simulink model "c6_p8x"  (Simulink 7.4)
settings: Solver=ode45  StartTime=0.0  StopTime=10e-6  MaxStep=0.1e-9  RelTol=1e-3
StopFcn:
  | plot_spar(spar)
undefined symbols (not defined in the file or in its folder): magnitude
libraries: powerlib x41, dspindex x12, dspsigops x6, dspbuff3 x4, dspxfrm3 x4, dsparch3 x4, dsparch4 x4, dspsnks4 x2, dspmtrx3 x2, simulink x1
settings Model: Creator=dbenson  LastModifiedBy=Dick
settings OptimizationCC: InlineInvariantSignals=on  InitFltsAndDblsToZero=on
settings DebuggingCC: SaveWithParameterizedLinksMsg=none  SignalResolutionControl=TryResolveAllWithWarning  MultiTaskDSMMsg=warning  MultiTaskCondExecSysMsg=none  StrictBusMsg=None
settings RTWCC: IncludeERTFirstTime=on
settings GRTTargetCC: TargetFcnLib=ansi_tfl_tmw.mat

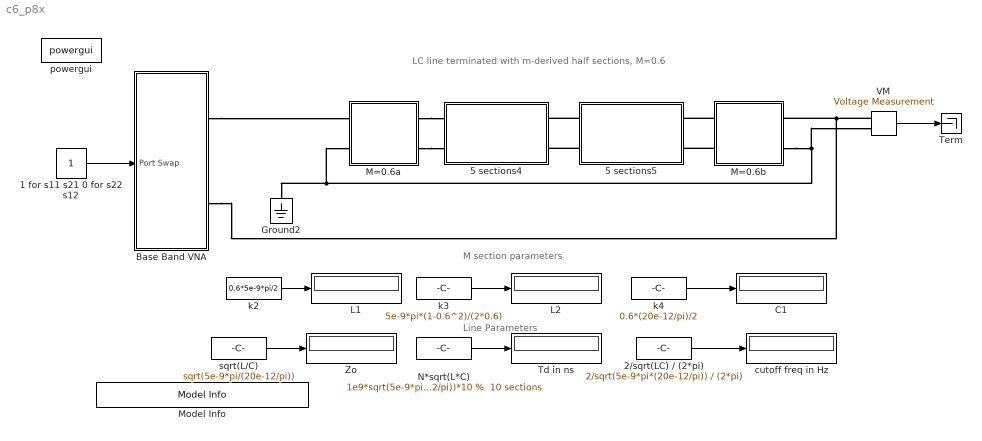
== system c6_p8x ==
  note: LC line terminated with m-derived half sections, M=0.6
  note: Line Parameters
  note: M section parameters
  1 for s11 s21 0 for s22 s12 : Constant  OutDataType=fixdt(1, 16)  OutScaling=2^0
  2/sqrt(LC) / (2*pi) : Constant  Value=2/sqrt(5e-9*pi*(20e-12/pi)) / (2*pi)  OutDataType=sfix(16)  OutScaling=2^0
  5 sections4 : Subsystem
  5 sections5 : Subsystem
  Base Band VNA : Subsystem  Description=Spectrum Analyzer  mask{BW=1e9, Frame_Size=512}
      mask prompts: BW "Bandwidth"; Frame_Size "FFT SIze (256,512,1024 etc)"
  C1 : Display
  Ground2 : powerlib/Elements/Ground  DialogController=POWERSYS.PowerSysDialog  PhysicalDomain=powersysdomain  SubClassName=unknown  LeftPortType=p1  RightPortType=p1  LConnTagsString=a
  L1 : Display
  L2 : Display
  M=0.6a : Subsystem
  M=0.6b : Subsystem
  Model Info : simulink/Model-Wide Utilities/Model Info  SystemSampleTime=-1  InitialBlockCM=None  BlockCM=None  Frame=on  DisplayStringWithTags=Copywrite 2005-2010 The MathWorks, Inc.  HorizontalTextAlignment=Center  LeftAlignmentValue=0.5  SourceBlockDiagram=c6_p8x  TagMaxNumber=20
  N*sqrt(L*C) : Constant  Value="1e9*sqrt(5e-9*pi*(20e-12/pi))*10 %  10 sections"  OutDataType=sfix(16)  OutScaling=2^0
  Td in ns : Display
  Term : Terminator
  VM : powerlib/Measurements/Voltage Measurement  DialogController=POWERSYS.PowerSysDialog  SystemSampleTime=-1  PhasorSimulation=off  OutputType=Complex  PSBequivalent=0
  Zo : Display
  cutoff freq in Hz : Display
  k2 : Constant  Value=0.6*5e-9*pi/2  OutDataType=sfix(16)  OutScaling=2^0
  k3 : Constant  Value=5e-9*pi*(1-0.6^2)/(2*0.6)  OutDataType=sfix(16)  OutScaling=2^0
  k4 : Constant  Value=0.6*(20e-12/pi)/2  OutDataType=sfix(16)  OutScaling=2^0
  powergui : powerlib/powergui  SystemSampleTime=-1  SimulationMode=Continuous  SampleTime=50e-6  frequency=60  SPID=off  DisableSnubberDevices=off  DisableRonSwitches=off  DisableVfSwitches=off  SwTol=0  Interpol=off  frequencyindice=0  echomessages=off  HookPort=off  DisplayEquations=off  FunctionMessages=off  EnableUseOfTLC=off  x0status=blocks  RestoreLinks=warning  Frange=[0:2:500]  Ylog=off  Xlog=on  ShowGrid=off  save=off  variable=ZData  ZoomFFT=on  StartTime=0.0  cycles=1  DisplayStyle=1  fundamental=60  FreqAxis=off  MaxFrequency=1000  frequencyindicesteady=1  RmsSteady=1  display=off  Ts=0  methode=off
  sqrt(L/C) : Constant  Value=sqrt(5e-9*pi/(20e-12/pi))  OutDataType=sfix(16)  OutScaling=2^0
  wires:
  sqrt(L/C)/1 -> Zo/1
  N*sqrt(L*C)/1 -> Td in ns/1
  k2/1 -> L1/1
  k3/1 -> L2/1
  k4/1 -> C1/1
  2/sqrt(LC) / (2*pi)/1 -> cutoff freq in Hz/1
  VM/1 -> Term/1
  1 for s11 s21 0 for s22 s12/1 -> Base Band VNA/1(Port Swap)
  connections:
  VM/LConn1 -- M=0.6b/RConn1 -- Base Band VNA/RConn2
  M=0.6a/RConn2 -- 5 sections4/LConn2
  5 sections5/LConn1 -- 5 sections4/RConn1
  5 sections5/LConn2 -- 5 sections4/RConn2
  M=0.6b/LConn1 -- 5 sections5/RConn1
  M=0.6b/LConn2 -- 5 sections5/RConn2
  M=0.6a/RConn1 -- 5 sections4/LConn1
  M=0.6b/RConn2 -- Ground2/LConn1 -- M=0.6a/LConn2 -- VM/LConn2
  Base Band VNA/RConn1 -- M=0.6a/LConn1

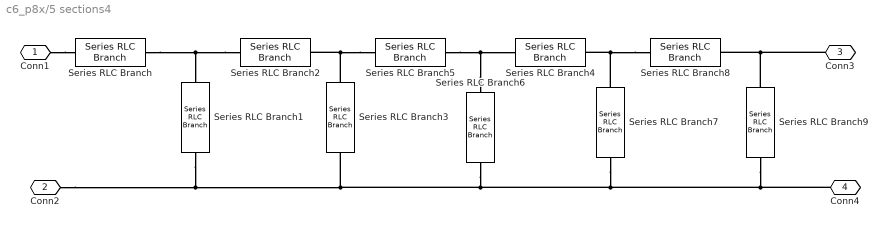
== system c6_p8x/5 sections4 ==
  Series RLC Branch{,2,4..5,8} (5 alike) : powerlib/Elements/Series RLC Branch  DialogController=POWERSYS.PowerSysDialog  PhysicalDomain=powersysdomain  SubClassName=unknown  LeftPortType=p1  RightPortType=p1  LConnTagsString=__new0  RConnTagsString=__new0  BranchType=L  Resistance=1.0  Inductance=5*pi*1e-9  SetiL0=off  InitialCurrent=0  Capacitance=1.0  Setx0=off  InitialVoltage=0  Measurements=None
  Series RLC Branch{1,3,6..7,9} (5 alike) : powerlib/Elements/Series RLC Branch  DialogController=POWERSYS.PowerSysDialog  PhysicalDomain=powersysdomain  SubClassName=unknown  LeftPortType=p1  RightPortType=p1  LConnTagsString=__new0  RConnTagsString=__new0  BranchType=C  Resistance=1.0  Inductance=1.0  SetiL0=off  InitialCurrent=0  Capacitance=20e-12/pi  Setx0=off  InitialVoltage=0  Measurements=None
  Conn1 : PMIOPort  Port=1  Side=Left
  Conn2 : PMIOPort  Port=2  Side=Left
  Conn3 : PMIOPort  Port=3  Side=Right
  Conn4 : PMIOPort  Port=4  Side=Right
  connections:
  Conn1/RConn1 -- Series RLC Branch/LConn1
  Conn3/RConn1 -- Series RLC Branch8/RConn1 -- Series RLC Branch9/LConn1
  Series RLC Branch8/LConn1 -- Series RLC Branch4/RConn1 -- Series RLC Branch7/LConn1
  Series RLC Branch6/LConn1 -- Series RLC Branch4/LConn1 -- Series RLC Branch5/RConn1
  Series RLC Branch5/LConn1 -- Series RLC Branch2/RConn1 -- Series RLC Branch3/LConn1
  Series RLC Branch7/RConn1 -- Conn4/RConn1 -- Series RLC Branch9/RConn1 -- Conn2/RConn1 -- Series RLC Branch1/RConn1 -- Series RLC Branch3/RConn1 -- Series RLC Branch6/RConn1
  Series RLC Branch2/LConn1 -- Series RLC Branch1/LConn1 -- Series RLC Branch/RConn1

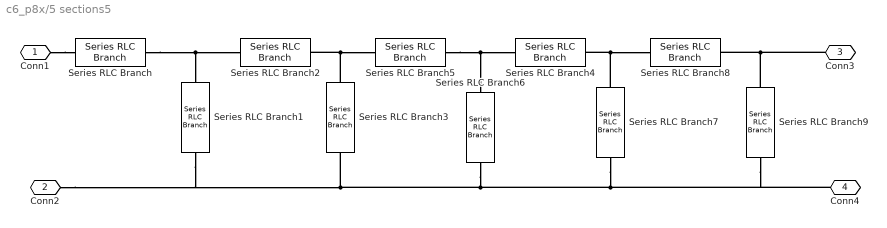
== system c6_p8x/5 sections5 ==
  Series RLC Branch{,2,4..5,8} (5 alike) : powerlib/Elements/Series RLC Branch  DialogController=POWERSYS.PowerSysDialog  PhysicalDomain=powersysdomain  SubClassName=unknown  LeftPortType=p1  RightPortType=p1  LConnTagsString=__new0  RConnTagsString=__new0  BranchType=L  Resistance=1.0  Inductance=5*pi*1e-9  SetiL0=off  InitialCurrent=0  Capacitance=1.0  Setx0=off  InitialVoltage=0  Measurements=None
  Series RLC Branch{1,3,6..7,9} (5 alike) : powerlib/Elements/Series RLC Branch  DialogController=POWERSYS.PowerSysDialog  PhysicalDomain=powersysdomain  SubClassName=unknown  LeftPortType=p1  RightPortType=p1  LConnTagsString=__new0  RConnTagsString=__new0  BranchType=C  Resistance=1.0  Inductance=1.0  SetiL0=off  InitialCurrent=0  Capacitance=20e-12/pi  Setx0=off  InitialVoltage=0  Measurements=None
  Conn1 : PMIOPort  Port=1  Side=Left
  Conn2 : PMIOPort  Port=2  Side=Left
  Conn3 : PMIOPort  Port=3  Side=Right
  Conn4 : PMIOPort  Port=4  Side=Right
  connections:
  Series RLC Branch/RConn1 -- Series RLC Branch1/LConn1 -- Series RLC Branch2/LConn1
  Series RLC Branch6/RConn1 -- Series RLC Branch3/RConn1 -- Series RLC Branch1/RConn1 -- Conn2/RConn1 -- Series RLC Branch9/RConn1 -- Conn4/RConn1 -- Series RLC Branch7/RConn1
  Series RLC Branch3/LConn1 -- Series RLC Branch2/RConn1 -- Series RLC Branch5/LConn1
  Series RLC Branch5/RConn1 -- Series RLC Branch4/LConn1 -- Series RLC Branch6/LConn1
  Series RLC Branch7/LConn1 -- Series RLC Branch4/RConn1 -- Series RLC Branch8/LConn1
  Series RLC Branch9/LConn1 -- Series RLC Branch8/RConn1 -- Conn3/RConn1
  Conn1/RConn1 -- Series RLC Branch/LConn1

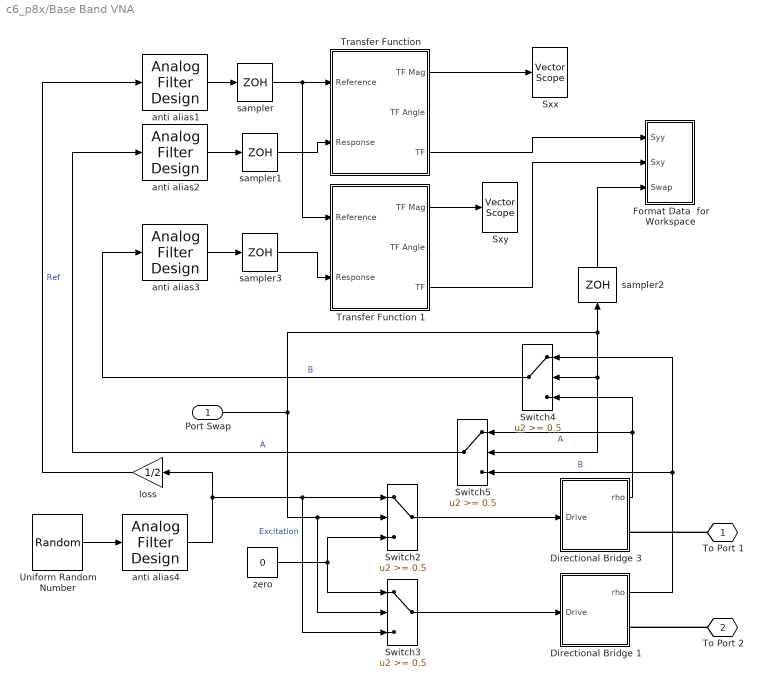
== system c6_p8x/Base Band VNA ==
  Port Swap : Inport  OutDataType=sfix(16)  OutScaling=2^0
  Directional Bridge 1 : Subsystem  mask{Zo=50}
      mask prompts: Zo "Zo="
  Directional Bridge 3 : Subsystem  mask{Zo=50}
      mask prompts: Zo "Zo="
  Format Data  for Workspace : Subsystem
  Switch{2..5} (4 alike) : Switch  Threshold=0.5  SaturateOnIntegerOverflow=on
  Sxx : dspsnks4/Vector Scope  DialogController=dspdialog.VectorScope  DialogControllerArgs=DataTag0  ScopeProperties=on  Domain=Frequency  HorizSpan=1  DisplayProperties=off  AxisGrid=on  Memory=off  FrameNumber=on  AxisLegend=off  AxisZoom=off  OpenScopeAtSimStart=on  OpenScopeImmediately=off  FigPos=[396 210 335 234]  AxisProperties=off  XUnits=Hertz  XRange=[0...Fs/2]  InheritXIncr=off  XIncr=1/(2.56*BW)  XLabel=Time  XLimit=Auto  XMin=0  XMax=1  XStart=0  YUnits=dB  YLabel=Amplitude  LineProperties=off  XAxisParamsVer=6.9
      settings: YMin=-30  YMax=25
  Sxy : dspsnks4/Vector Scope  DialogController=dspdialog.VectorScope  DialogControllerArgs=DataTag1  ScopeProperties=on  Domain=Frequency  HorizSpan=1  DisplayProperties=off  AxisGrid=on  Memory=off  FrameNumber=on  AxisLegend=off  AxisZoom=off  OpenScopeAtSimStart=on  OpenScopeImmediately=off  FigPos=[24 215 357 231]  AxisProperties=off  XUnits=Hertz  XRange=[0...Fs/2]  InheritXIncr=off  XIncr=1/(2.56*BW)  XLabel=Time  XLimit=Auto  XMin=0  XMax=1  XStart=0  YUnits=dB  YLabel=Amplitude  LineProperties=off  XAxisParamsVer=6.9
      settings: YMin=-30  YMax=25
  "Transfer Function " : Subsystem  mask{NFFT=Frame_Size, Navg=100, pcnt=100, unwrap_flag=on}
      mask prompts: NFFT "FFT length (power of 2):"; Navg "Spectral Averaging Factor (>=1):"; pcnt "Percentage of  Alias Free Data  (<=100)"; unwrap_flag "Unwrap Phase"
      mask Display: disp('Transfer Function \n Estimation (v2.0) ')
  Transfer Function 1 : Subsystem  mask{NFFT=Frame_Size, Navg=100, pcnt=100, unwrap_flag=on}
      mask prompts: NFFT "FFT length (power of 2):"; Navg "Spectral Averaging Factor (>=1):"; pcnt "Percentage of  Alias Free Data  (<=100)"; unwrap_flag "Unwrap Phase"
      mask Display: disp('Transfer Function \n Estimation (v2.0) ')
  Uniform Random Number : UniformRandomNumber  SampleTime=1/(2.56*BW)
  anti alias{1..4} (4 alike) : dsparch4/Analog Filter Design  method=Elliptic  filttype=Lowpass  N=8  Wlo=BW*2*pi  Whi=80  Rp=2  Rs=100
  loss : Gain  Gain=1/2  ParameterDataType=sfix(16)  ParameterScaling=2^0  OutDataType=sfix(16)  OutScaling=2^0  SaturateOnIntegerOverflow=on  OutDataTypeStr=Inherit: Same as input  ParamDataTypeStr=Inherit: Same as input
  sampler : ZeroOrderHold  SampleTime=1/(2.56*BW)
  sampler1 : ZeroOrderHold  SampleTime=1/(2.56*BW)
  sampler2 : ZeroOrderHold  SampleTime=256/(2.56*BW)
  sampler3 : ZeroOrderHold  SampleTime=1/(2.56*BW)
  zero : Constant  Value=0  OutDataType=sfix(16)  OutScaling=2^0
  To Port 1 : PMIOPort  Tag=PMCPort  Port=1  Side=Right
  To Port 2 : PMIOPort  Tag=PMCPort  Port=2  Side=Right
  wires:
  sampler/1 -> "Transfer Function "/1(Reference), Transfer Function 1/1(Reference)
  anti alias1/1 -> sampler/1
  anti alias2/1 -> sampler1/1
  Uniform Random Number/1 -> anti alias4/1
  anti alias3/1 -> sampler3/1
  sampler3/1 -> Transfer Function 1/2(Response)
  anti alias4/1 -> loss/1, Switch3/3, Switch2/1  "Excitation"
  loss/1 -> anti alias1/1  "Ref"
  Port Swap/1 -> Switch3/2, Switch2/2, Switch4/2, Switch5/2, sampler2/1
  zero/1 -> Switch2/3, Switch3/1
  Switch2/1 -> Directional Bridge 3/1(Drive)
  Switch3/1 -> Directional Bridge 1/1(Drive)
  Switch5/1 -> anti alias2/1  "A"
  Switch4/1 -> anti alias3/1  "B"
  Directional Bridge 3/1(rho) -> Switch4/3, Switch5/1  "A"
  Directional Bridge 1/1(rho) -> Switch5/3, Switch4/1  "B"
  sampler1/1 -> "Transfer Function "/2(Response)
  "Transfer Function "/1(TF Mag) -> Sxx/1
  Transfer Function 1/3("TF ") -> Format Data  for Workspace/2(Sxy)
  Transfer Function 1/1(TF Mag) -> Sxy/1
  "Transfer Function "/3("TF ") -> Format Data  for Workspace/1(Syy)
  sampler2/1 -> Format Data  for Workspace/3(Swap)
  connections:
  To Port 1/RConn1 -- Directional Bridge 3/RConn1
  To Port 2/RConn1 -- Directional Bridge 1/RConn1

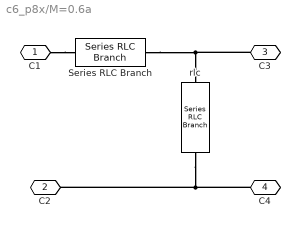
== system c6_p8x/M=0.6a ==
  Series RLC Branch : powerlib/Elements/Series RLC Branch  DialogController=POWERSYS.PowerSysDialog  PhysicalDomain=powersysdomain  SubClassName=unknown  LeftPortType=p1  RightPortType=p1  LConnTagsString=__new0  RConnTagsString=__new0  BranchType=L  Resistance=1.0  Inductance=4.712e-9  SetiL0=off  InitialCurrent=0  Capacitance=1.0  Setx0=off  InitialVoltage=0  Measurements=None
  rlc : powerlib/Elements/Series RLC Branch  DialogController=POWERSYS.PowerSysDialog  PhysicalDomain=powersysdomain  SubClassName=unknown  LeftPortType=p1  RightPortType=p1  LConnTagsString=__new0  RConnTagsString=__new0  BranchType=LC  Resistance=1.0  Inductance=8.378e-9  SetiL0=off  InitialCurrent=0  Capacitance=1.91e-12  Setx0=off  InitialVoltage=0  Measurements=None
  C1 : PMIOPort  Port=1  Side=Left
  C2 : PMIOPort  Port=2  Side=Left
  C3 : PMIOPort  Port=3  Side=Right
  C4 : PMIOPort  Port=4  Side=Right
  connections:
  C3/RConn1 -- rlc/LConn1 -- Series RLC Branch/RConn1
  C4/RConn1 -- C2/RConn1 -- rlc/RConn1
  C1/RConn1 -- Series RLC Branch/LConn1

== system c6_p8x/M=0.6b ==
  Series RLC Branch : powerlib/Elements/Series RLC Branch  DialogController=POWERSYS.PowerSysDialog  PhysicalDomain=powersysdomain  SubClassName=unknown  LeftPortType=p1  RightPortType=p1  LConnTagsString=__new0  RConnTagsString=__new0  BranchType=L  Resistance=1.0  Inductance=4.712e-9  SetiL0=off  InitialCurrent=0  Capacitance=1.0  Setx0=off  InitialVoltage=0  Measurements=None
  rlc : powerlib/Elements/Series RLC Branch  DialogController=POWERSYS.PowerSysDialog  PhysicalDomain=powersysdomain  SubClassName=unknown  LeftPortType=p1  RightPortType=p1  LConnTagsString=__new0  RConnTagsString=__new0  BranchType=LC  Resistance=1.0  Inductance=8.378e-9  SetiL0=off  InitialCurrent=0  Capacitance=1.91e-12  Setx0=off  InitialVoltage=0  Measurements=None
  C1 : PMIOPort  Port=1  Side=Left
  C2 : PMIOPort  Port=2  Side=Left
  C3 : PMIOPort  Port=3  Side=Right
  C4 : PMIOPort  Port=4  Side=Right
  connections:
  C1/RConn1 -- Series RLC Branch/LConn1
  rlc/RConn1 -- C2/RConn1 -- C4/RConn1
  Series RLC Branch/RConn1 -- rlc/LConn1 -- C3/RConn1

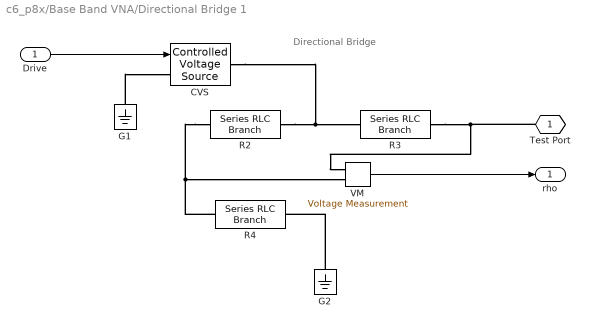
== system c6_p8x/Base Band VNA/Directional Bridge 1 ==
  note: Directional Bridge
  Drive : Inport  OutDataType=sfix(16)  OutScaling=2^0
  CVS : powerlib/Electrical Sources/Controlled Voltage Source  Description=source block  DialogController=POWERSYS.PowerSysDialog  SystemSampleTime=-1  Initialize=off  Source_Type=AC  Amplitude=0  Phase=0  Frequency=0  Measurements=None
      settings: AttributesFormatString=\n
  G1 : powerlib/Elements/Ground  DialogController=POWERSYS.PowerSysDialog  PhysicalDomain=powersysdomain  SubClassName=unknown  LeftPortType=p1  RightPortType=p1  LConnTagsString=a
  G2 : powerlib/Elements/Ground  DialogController=POWERSYS.PowerSysDialog  PhysicalDomain=powersysdomain  SubClassName=unknown  LeftPortType=p1  RightPortType=p1  LConnTagsString=a
  R2 : powerlib/Elements/Series RLC Branch  DialogController=POWERSYS.PowerSysDialog  PhysicalDomain=powersysdomain  SubClassName=unknown  LeftPortType=p1  RightPortType=p1  LConnTagsString=__new0  RConnTagsString=__new0  BranchType=R  Resistance=Zo  Inductance=1.0  SetiL0=off  InitialCurrent=0  Capacitance=1.0  Setx0=off  InitialVoltage=0  Measurements=None
  R3 : powerlib/Elements/Series RLC Branch  DialogController=POWERSYS.PowerSysDialog  PhysicalDomain=powersysdomain  SubClassName=unknown  LeftPortType=p1  RightPortType=p1  LConnTagsString=__new0  RConnTagsString=__new0  BranchType=R  Resistance=Zo  Inductance=1.0  SetiL0=off  InitialCurrent=0  Capacitance=1.0  Setx0=off  InitialVoltage=0  Measurements=None
  R4 : powerlib/Elements/Series RLC Branch  DialogController=POWERSYS.PowerSysDialog  PhysicalDomain=powersysdomain  SubClassName=unknown  LeftPortType=p1  RightPortType=p1  LConnTagsString=__new0  RConnTagsString=__new0  BranchType=R  Resistance=Zo  Inductance=1.0  SetiL0=off  InitialCurrent=0  Capacitance=1.0  Setx0=off  InitialVoltage=0  Measurements=None
  VM : powerlib/Measurements/Voltage Measurement  Tag=PoWeRsYsTeMmEaSuReMeNt  DialogController=POWERSYS.PowerSysDialog  SystemSampleTime=-1  PhasorSimulation=off  OutputType=Magnitude  PSBequivalent=0
  Test Port : PMIOPort  Tag=PMCPort  Port=1  Side=Right
  rho : Outport  OutDataType=sfix(16)  OutScaling=2^0
  wires:
  Drive/1 -> CVS/1
  VM/1 -> rho/1
  connections:
  G1/LConn1 -- CVS/LConn1
  Test Port/RConn1 -- VM/LConn1 -- R3/RConn1
  G2/LConn1 -- R4/RConn1
  R2/LConn1 -- VM/LConn2 -- R4/LConn1
  CVS/RConn1 -- R3/LConn1 -- R2/RConn1

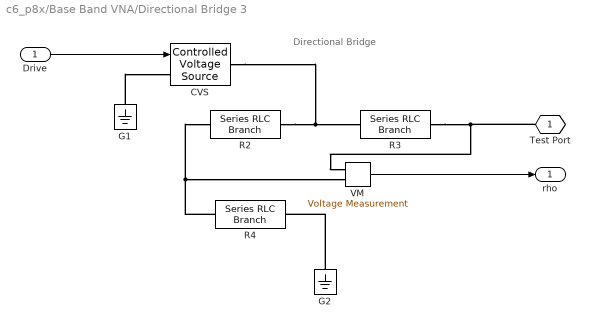
== system c6_p8x/Base Band VNA/Directional Bridge 3 ==
  note: Directional Bridge
  Drive : Inport  OutDataType=sfix(16)  OutScaling=2^0
  CVS : powerlib/Electrical Sources/Controlled Voltage Source  Description=source block  DialogController=POWERSYS.PowerSysDialog  SystemSampleTime=-1  Initialize=off  Source_Type=AC  Amplitude=0  Phase=0  Frequency=0  Measurements=None
      settings: AttributesFormatString=\n
  G1 : powerlib/Elements/Ground  DialogController=POWERSYS.PowerSysDialog  PhysicalDomain=powersysdomain  SubClassName=unknown  LeftPortType=p1  RightPortType=p1  LConnTagsString=a
  G2 : powerlib/Elements/Ground  DialogController=POWERSYS.PowerSysDialog  PhysicalDomain=powersysdomain  SubClassName=unknown  LeftPortType=p1  RightPortType=p1  LConnTagsString=a
  R2 : powerlib/Elements/Series RLC Branch  DialogController=POWERSYS.PowerSysDialog  PhysicalDomain=powersysdomain  SubClassName=unknown  LeftPortType=p1  RightPortType=p1  LConnTagsString=__new0  RConnTagsString=__new0  BranchType=R  Resistance=Zo  Inductance=1.0  SetiL0=off  InitialCurrent=0  Capacitance=1.0  Setx0=off  InitialVoltage=0  Measurements=None
  R3 : powerlib/Elements/Series RLC Branch  DialogController=POWERSYS.PowerSysDialog  PhysicalDomain=powersysdomain  SubClassName=unknown  LeftPortType=p1  RightPortType=p1  LConnTagsString=__new0  RConnTagsString=__new0  BranchType=R  Resistance=Zo  Inductance=1.0  SetiL0=off  InitialCurrent=0  Capacitance=1.0  Setx0=off  InitialVoltage=0  Measurements=None
  R4 : powerlib/Elements/Series RLC Branch  DialogController=POWERSYS.PowerSysDialog  PhysicalDomain=powersysdomain  SubClassName=unknown  LeftPortType=p1  RightPortType=p1  LConnTagsString=__new0  RConnTagsString=__new0  BranchType=R  Resistance=Zo  Inductance=1.0  SetiL0=off  InitialCurrent=0  Capacitance=1.0  Setx0=off  InitialVoltage=0  Measurements=None
  VM : powerlib/Measurements/Voltage Measurement  Tag=PoWeRsYsTeMmEaSuReMeNt  DialogController=POWERSYS.PowerSysDialog  SystemSampleTime=-1  PhasorSimulation=off  OutputType=Magnitude  PSBequivalent=0
  Test Port : PMIOPort  Tag=PMCPort  Port=1  Side=Right
  rho : Outport  OutDataType=sfix(16)  OutScaling=2^0
  wires:
  VM/1 -> rho/1
  Drive/1 -> CVS/1
  connections:
  R2/RConn1 -- R3/LConn1 -- CVS/RConn1
  R4/LConn1 -- VM/LConn2 -- R2/LConn1
  G2/LConn1 -- R4/RConn1
  R3/RConn1 -- VM/LConn1 -- Test Port/RConn1
  G1/LConn1 -- CVS/LConn1

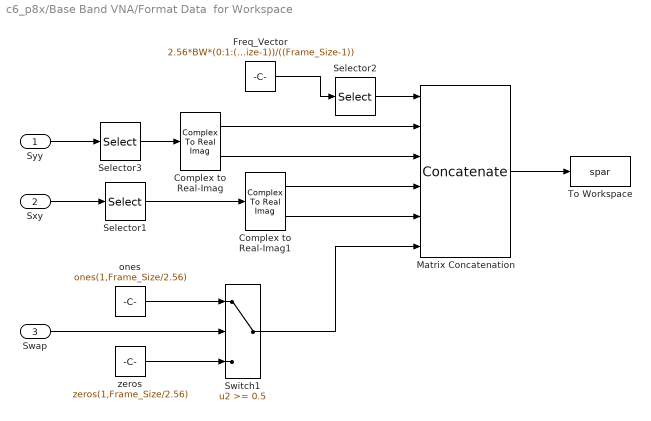
== system c6_p8x/Base Band VNA/Format Data  for Workspace ==
  Syy : Inport  OutDataType=sfix(16)  OutScaling=2^0
  Sxy : Inport  Port=2  OutDataType=sfix(16)  OutScaling=2^0
  Swap : Inport  Port=3  OutDataType=sfix(16)  OutScaling=2^0
  Complex to Real-Imag : ComplexToRealImag
  Complex to Real-Imag1 : ComplexToRealImag
  Freq_Vector : Constant  Value=2.56*BW*(0:1:(Frame_Size-1))/((Frame_Size-1))  OutDataType=sfix(16)  OutScaling=2^0
  Matrix Concatenation : Concatenate  NumInputs=6  Mode=Multidimensional array  ConcatenateDimension=2
  Selector1 : Selector  InputPortWidth=Frame_Size  IndexOptions=Index vector (dialog)  Indices=[1:Frame_Size/2.56]  OutputSizes=1
  Selector2 : Selector  InputPortWidth=Frame_Size  IndexOptions=Index vector (dialog)  Indices=[1:Frame_Size/2.56]  OutputSizes=1
  Selector3 : Selector  InputPortWidth=Frame_Size  IndexOptions=Index vector (dialog)  Indices=[1:Frame_Size/2.56]  OutputSizes=1
  Switch1 : Switch  Threshold=0.5  SaturateOnIntegerOverflow=on
  To Workspace : ToWorkspace  VariableName=spar  SampleTime=-1  SaveFormat=Array
      settings: MaxDataPoints=1
  ones : Constant  Value=ones(1,Frame_Size/2.56)  OutDataType=sfix(16)  OutScaling=2^0
  zeros : Constant  Value=zeros(1,Frame_Size/2.56)  OutDataType=sfix(16)  OutScaling=2^0
  wires:
  Matrix Concatenation/1 -> To Workspace/1
  Complex to Real-Imag1/2 -> Matrix Concatenation/5
  Freq_Vector/1 -> Selector2/1
  Complex to Real-Imag/1 -> Matrix Concatenation/2
  Complex to Real-Imag/2 -> Matrix Concatenation/3
  Complex to Real-Imag1/1 -> Matrix Concatenation/4
  Syy/1 -> Selector3/1
  Sxy/1 -> Selector1/1
  ones/1 -> Switch1/1
  zeros/1 -> Switch1/3
  Swap/1 -> Switch1/2
  Switch1/1 -> Matrix Concatenation/6
  Selector3/1 -> Complex to Real-Imag/1
  Selector1/1 -> Complex to Real-Imag1/1
  Selector2/1 -> Matrix Concatenation/1

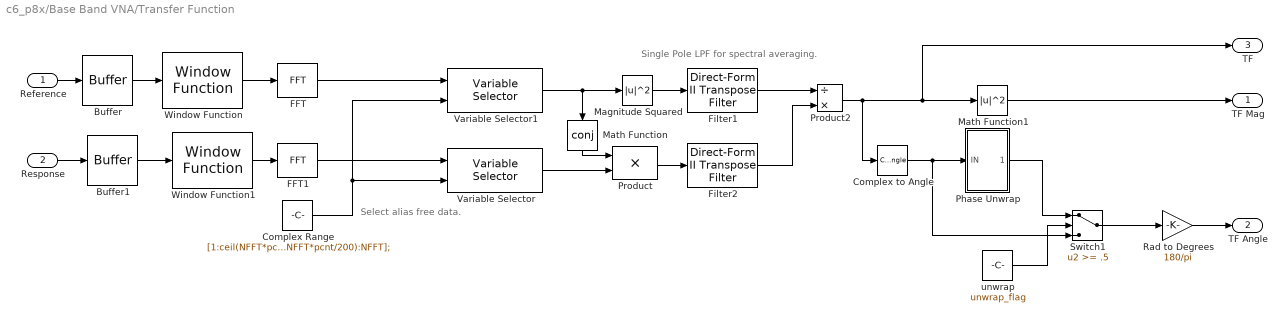
== system c6_p8x/Base Band VNA/Transfer Function  ==
  note: Select alias free data.
  note: Single Pole LPF for spectral averaging.
  Reference : Inport  OutDataType=sfix(16)  OutScaling=2^0
  Response : Inport  Port=2  OutDataType=sfix(16)  OutScaling=2^0
  Buffer : dspbuff3/Buffer  N=NFFT  V=0  ic=0
  Buffer1 : dspbuff3/Buffer  N=NFFT  V=0  ic=0
  Complex Range : Constant  Value=[1:ceil(NFFT*pcnt/200),ceil(1+NFFT-NFFT*pcnt/200):NFFT];  OutDataType=sfix(16)  OutScaling=2^0
  Complex to Angle : ComplexToMagnitudeAngle  Output=Angle
  FFT : dspxfrm3/FFT  DialogController=dspDDGCreate  DialogControllerArgs=DataTag2  CompMethod=Table lookup  TableOpt=NEW  TableOptActive=Speed  BitRevOrder=off  InheritFFTLength=on  FFTLength=64  SkipNorm=on  firstCoeffMode=Specify word length  firstCoeffWordLength=16  firstCoeffFracLength=15  roundingMode=Floor  overflowMode=off
  FFT1 : dspxfrm3/FFT  DialogController=dspDDGCreate  DialogControllerArgs=DataTag3  CompMethod=Table lookup  TableOpt=NEW  TableOptActive=Speed  BitRevOrder=off  InheritFFTLength=on  FFTLength=64  SkipNorm=on  firstCoeffMode=User-defined  firstCoeffWordLength=16  firstCoeffFracLength=15  roundingMode=Floor  overflowMode=off
  Filter1 : dsparch3/Direct-Form II Transpose Filter  num=1  den=[Navg -(Navg-1)]  ic=eps
  Filter2 : dsparch3/Direct-Form II Transpose Filter  num=1  den=[Navg -(Navg-1)]  ic=eps
  Magnitude Squared : Math  Operator=magnitude^2  OutDataType=sfix(16)  OutScaling=2^0  SaturateOnIntegerOverflow=on
  Math Function : Math  Operator=conj  OutDataType=sfix(16)  OutScaling=2^0  SaturateOnIntegerOverflow=on
  Math Function1 : Math  Operator=magnitude^2  OutDataType=sfix(16)  OutScaling=2^0  SaturateOnIntegerOverflow=on
  Phase Unwrap : Subsystem
  Product : Product  OutDataType=sfix(16)  OutScaling=2^0  SaturateOnIntegerOverflow=on  InputSameDT=on  OutDataTypeStr=Inherit: Same as first input
  Product2 : Product  Inputs=/*  OutDataType=sfix(16)  OutScaling=2^0  SaturateOnIntegerOverflow=on  InputSameDT=on  OutDataTypeStr=Inherit: Same as first input
  Rad to Degrees : Gain  Gain=180/pi  ParameterDataType=sfix(16)  ParameterScaling=2^0  OutDataType=sfix(16)  OutScaling=2^0
  Switch1 : Switch  Threshold=.5
  Variable Selector : dspindex/Variable Selector  NumInputs=1  rowsOrCols=Rows  IdxMode=Variable  Elements=[1 3]  ZerOneIdxMode=One-based  errmode=Clip Index  FillMode=on  FillValues=0
  Variable Selector1 : dspindex/Variable Selector  NumInputs=1  rowsOrCols=Rows  IdxMode=Variable  Elements=[1 3]  ZerOneIdxMode=One-based  errmode=Clip Index  FillMode=on  FillValues=0
  Window Function : dspsigops/Window Function  DialogController=dspDDGCreate  DialogControllerArgs=DataTag5  winmode=Apply window to input  wintype=Hann  sampmode=Continuous  samptime=1  N=64  Rs=50  beta=10  winsamp=Periodic  UserWindow=hamming  OptParams=off  UserParams={'symmetric'}  dataType=double  isSigned=on  wordLen=16  udDataType=sfix(16)  fracBitsMode=Best precision  numFracBits=15  roundingMode=Floor  overflowMode=off  numSidelobes=4  sidelobeLevel=-30
  Window Function1 : dspsigops/Window Function  DialogController=dspDDGCreate  DialogControllerArgs=DataTag6  winmode=Apply window to input  wintype=Hann  sampmode=Continuous  samptime=1  N=64  Rs=50  beta=10  winsamp=Periodic  UserWindow=hamming  OptParams=off  UserParams={'symmetric'}  dataType=double  isSigned=on  wordLen=16  udDataType=sfix(16)  fracBitsMode=Best precision  numFracBits=15  roundingMode=Floor  overflowMode=off  numSidelobes=4  sidelobeLevel=-30
  unwrap : Constant  Value=unwrap_flag  OutDataType=sfix(16)  OutScaling=2^0
  TF Mag : Outport  OutDataType=sfix(16)  OutScaling=2^0
  TF Angle : Outport  Port=2  OutDataType=sfix(16)  OutScaling=2^0
  "TF " : Outport  Port=3  OutDataType=sfix(16)  OutScaling=2^0
  wires:
  Phase Unwrap/1(Out1) -> Switch1/1
  unwrap/1 -> Switch1/2
  Switch1/1 -> Rad to Degrees/1
  Variable Selector1/1 -> Math Function/1, Magnitude Squared/1
  Variable Selector/1 -> Product/2
  Product2/1 -> Complex to Angle/1, Math Function1/1, "TF "/1
  Buffer1/1 -> Window Function1/1
  Buffer/1 -> Window Function/1
  Filter2/1 -> Product2/2
  Filter1/1 -> Product2/1
  Window Function1/1 -> FFT1/1
  Window Function/1 -> FFT/1
  Math Function1/1 -> TF Mag/1
  FFT/1 -> Variable Selector1/1
  Magnitude Squared/1 -> Filter1/1
  Math Function/1 -> Product/1
  FFT1/1 -> Variable Selector/1
  Product/1 -> Filter2/1
  Reference/1 -> Buffer/1
  Response/1 -> Buffer1/1
  Rad to Degrees/1 -> TF Angle/1
  Complex to Angle/1 -> Phase Unwrap/1(IN), Switch1/3
  Complex Range/1 -> Variable Selector1/2, Variable Selector/2

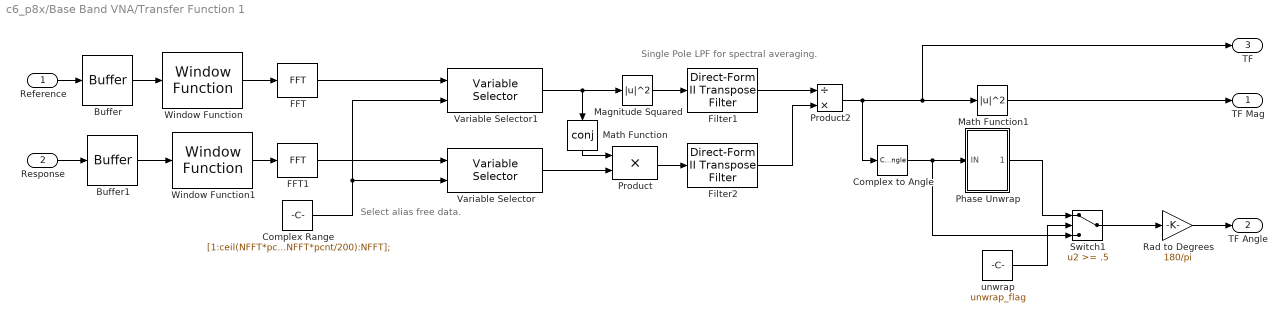
== system c6_p8x/Base Band VNA/Transfer Function 1 ==
  note: Single Pole LPF for spectral averaging.
  note: Select alias free data.
  Reference : Inport  OutDataType=sfix(16)  OutScaling=2^0
  Response : Inport  Port=2  OutDataType=sfix(16)  OutScaling=2^0
  Buffer : dspbuff3/Buffer  N=NFFT  V=0  ic=0
  Buffer1 : dspbuff3/Buffer  N=NFFT  V=0  ic=0
  Complex Range : Constant  Value=[1:ceil(NFFT*pcnt/200),ceil(1+NFFT-NFFT*pcnt/200):NFFT];  OutDataType=sfix(16)  OutScaling=2^0
  Complex to Angle : ComplexToMagnitudeAngle  Output=Angle
  FFT : dspxfrm3/FFT  DialogController=dspDDGCreate  DialogControllerArgs=DataTag7  CompMethod=Table lookup  TableOpt=NEW  TableOptActive=Speed  BitRevOrder=off  InheritFFTLength=on  FFTLength=64  SkipNorm=on  firstCoeffMode=Specify word length  firstCoeffWordLength=16  firstCoeffFracLength=15  roundingMode=Floor  overflowMode=off
  FFT1 : dspxfrm3/FFT  DialogController=dspDDGCreate  DialogControllerArgs=DataTag8  CompMethod=Table lookup  TableOpt=NEW  TableOptActive=Speed  BitRevOrder=off  InheritFFTLength=on  FFTLength=64  SkipNorm=on  firstCoeffMode=User-defined  firstCoeffWordLength=16  firstCoeffFracLength=15  roundingMode=Floor  overflowMode=off
  Filter1 : dsparch3/Direct-Form II Transpose Filter  num=1  den=[Navg -(Navg-1)]  ic=eps
  Filter2 : dsparch3/Direct-Form II Transpose Filter  num=1  den=[Navg -(Navg-1)]  ic=eps
  Magnitude Squared : Math  Operator=magnitude^2  OutDataType=sfix(16)  OutScaling=2^0  SaturateOnIntegerOverflow=on
  Math Function : Math  Operator=conj  OutDataType=sfix(16)  OutScaling=2^0  SaturateOnIntegerOverflow=on
  Math Function1 : Math  Operator=magnitude^2  OutDataType=sfix(16)  OutScaling=2^0  SaturateOnIntegerOverflow=on
  Phase Unwrap : Subsystem
  Product : Product  OutDataType=sfix(16)  OutScaling=2^0  SaturateOnIntegerOverflow=on  InputSameDT=on  OutDataTypeStr=Inherit: Same as first input
  Product2 : Product  Inputs=/*  OutDataType=sfix(16)  OutScaling=2^0  SaturateOnIntegerOverflow=on  InputSameDT=on  OutDataTypeStr=Inherit: Same as first input
  Rad to Degrees : Gain  Gain=180/pi  ParameterDataType=sfix(16)  ParameterScaling=2^0  OutDataType=sfix(16)  OutScaling=2^0
  Switch1 : Switch  Threshold=.5
  Variable Selector : dspindex/Variable Selector  NumInputs=1  rowsOrCols=Rows  IdxMode=Variable  Elements=[1 3]  ZerOneIdxMode=One-based  errmode=Clip Index  FillMode=on  FillValues=0
  Variable Selector1 : dspindex/Variable Selector  NumInputs=1  rowsOrCols=Rows  IdxMode=Variable  Elements=[1 3]  ZerOneIdxMode=One-based  errmode=Clip Index  FillMode=on  FillValues=0
  Window Function : dspsigops/Window Function  DialogController=dspDDGCreate  DialogControllerArgs=DataTag10  winmode=Apply window to input  wintype=Hann  sampmode=Continuous  samptime=1  N=64  Rs=50  beta=10  winsamp=Periodic  UserWindow=hamming  OptParams=off  UserParams={'symmetric'}  dataType=double  isSigned=on  wordLen=16  udDataType=sfix(16)  fracBitsMode=Best precision  numFracBits=15  roundingMode=Floor  overflowMode=off  numSidelobes=4  sidelobeLevel=-30
  Window Function1 : dspsigops/Window Function  DialogController=dspDDGCreate  DialogControllerArgs=DataTag11  winmode=Apply window to input  wintype=Hann  sampmode=Continuous  samptime=1  N=64  Rs=50  beta=10  winsamp=Periodic  UserWindow=hamming  OptParams=off  UserParams={'symmetric'}  dataType=double  isSigned=on  wordLen=16  udDataType=sfix(16)  fracBitsMode=Best precision  numFracBits=15  roundingMode=Floor  overflowMode=off  numSidelobes=4  sidelobeLevel=-30
  unwrap : Constant  Value=unwrap_flag  OutDataType=sfix(16)  OutScaling=2^0
  TF Mag : Outport  OutDataType=sfix(16)  OutScaling=2^0
  TF Angle : Outport  Port=2  OutDataType=sfix(16)  OutScaling=2^0
  "TF " : Outport  Port=3  OutDataType=sfix(16)  OutScaling=2^0
  wires:
  Complex Range/1 -> Variable Selector/2, Variable Selector1/2
  Complex to Angle/1 -> Switch1/3, Phase Unwrap/1(IN)
  Rad to Degrees/1 -> TF Angle/1
  Response/1 -> Buffer1/1
  Reference/1 -> Buffer/1
  Product/1 -> Filter2/1
  FFT1/1 -> Variable Selector/1
  Math Function/1 -> Product/1
  Magnitude Squared/1 -> Filter1/1
  FFT/1 -> Variable Selector1/1
  Math Function1/1 -> TF Mag/1
  Window Function/1 -> FFT/1
  Window Function1/1 -> FFT1/1
  Filter1/1 -> Product2/1
  Filter2/1 -> Product2/2
  Buffer/1 -> Window Function/1
  Buffer1/1 -> Window Function1/1
  Product2/1 -> "TF "/1, Math Function1/1, Complex to Angle/1
  Variable Selector/1 -> Product/2
  Variable Selector1/1 -> Magnitude Squared/1, Math Function/1
  Switch1/1 -> Rad to Degrees/1
  unwrap/1 -> Switch1/2
  Phase Unwrap/1(Out1) -> Switch1/1

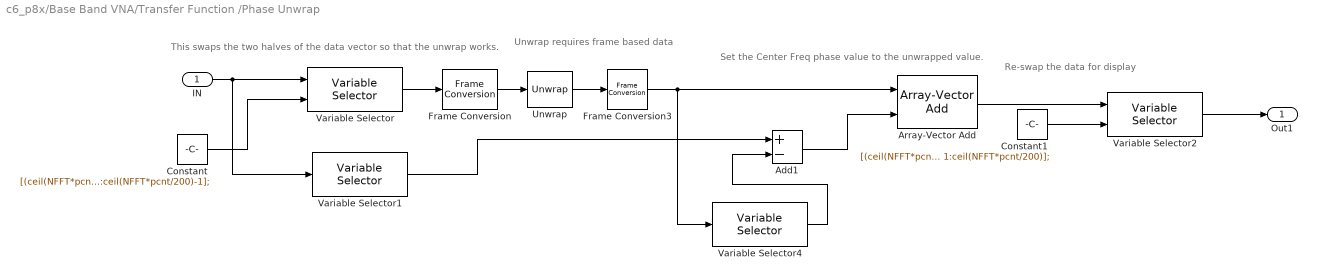
== system c6_p8x/Base Band VNA/Transfer Function /Phase Unwrap ==
  note: Unwrap requires frame based data
  note: Re-swap the data for display
  note: Set the Center Freq phase value to the unwrapped value.
  note: This swaps the two halves of the data vector
      | so that the unwrap works.
  IN : Inport  OutDataType=sfix(16)  OutScaling=2^0
  Add1 : Sum  Inputs=+-  OutDataType=sfix(16)  OutScaling=2^-10
  Array-Vector Add : dspmtrx3/Array-Vector Add  DialogController=dspDDGCreate  DialogControllerArgs=DataTag4  Dimension=2  V_Source=Input port  V_VectFromMask=[0.5 0.25]  firstCoeffDataTypeStr=Inherit: Same word length as input  firstCoeffLastDataTypeStr=Inherit: Same word length as input  firstCoeffMin=[]  firstCoeffMax=[]  outputDataTypeStr=Inherit: Same as accumulator  outputLastDataTypeStr=Inherit: Same as accumulator  outputMin=[]  outputMax=[]  roundingMode=Floor  overflowMode=off
  Constant : Constant  Value=[(ceil(NFFT*pcnt/200)):ceil(NFFT*pcnt/100) 1:ceil(NFFT*pcnt/200)-1];  OutDataType=sfix(16)  OutScaling=2^0
  Constant1 : Constant  Value=[(ceil(NFFT*pcnt/200)+1):ceil(NFFT*pcnt/100) 1:ceil(NFFT*pcnt/200)];  OutDataType=sfix(16)  OutScaling=2^0
  Frame Conversion : FrameConversion
  Frame Conversion3 : FrameConversion  OutFrame=Sample-based
  Unwrap : dspsigops/Unwrap  running=on  tol=pi
  Variable Selector : dspindex/Variable Selector  NumInputs=1  rowsOrCols=Rows  IdxMode=Variable  Elements=[1 3]  ZerOneIdxMode=One-based  errmode=Clip Index  FillMode=on  FillValues=0
  Variable Selector1 : dspindex/Variable Selector  NumInputs=1  rowsOrCols=Rows  IdxMode=Fixed  Elements=[1]  ZerOneIdxMode=One-based  errmode=Clip Index  FillMode=on  FillValues=0
  Variable Selector2 : dspindex/Variable Selector  NumInputs=1  rowsOrCols=Rows  IdxMode=Variable  Elements=[1 3]  ZerOneIdxMode=One-based  errmode=Clip Index  FillMode=on  FillValues=0
  Variable Selector4 : dspindex/Variable Selector  NumInputs=1  rowsOrCols=Rows  IdxMode=Fixed  Elements=length([(ceil(NFFT*pcnt/200)+1):ceil(NFFT*pcnt/100) 1:ceil(NFFT*pcnt/200)] )/2+1  ZerOneIdxMode=One-based  errmode=Clip Index  FillMode=on  FillValues=0
  Out1 : Outport  OutDataType=sfix(16)  OutScaling=2^0
  wires:
  Array-Vector Add/1 -> Variable Selector2/1
  Add1/1 -> Array-Vector Add/2
  Frame Conversion3/1 -> Array-Vector Add/1, Variable Selector4/1
  Constant1/1 -> Variable Selector2/2
  Variable Selector4/1 -> Add1/2
  Unwrap/1 -> Frame Conversion3/1
  Variable Selector1/1 -> Add1/1
  Variable Selector/1 -> Frame Conversion/1
  Constant/1 -> Variable Selector/2
  IN/1 -> Variable Selector1/1, Variable Selector/1
  Variable Selector2/1 -> Out1/1
  Frame Conversion/1 -> Unwrap/1

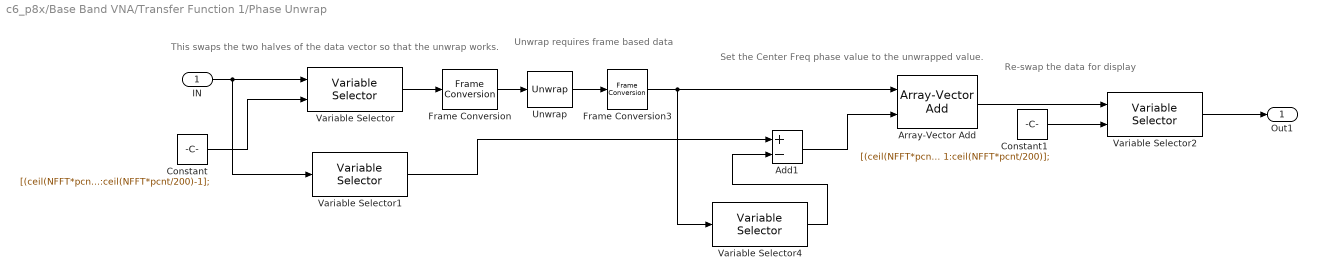
== system c6_p8x/Base Band VNA/Transfer Function 1/Phase Unwrap ==
  note: This swaps the two halves of the data vector
      | so that the unwrap works.
  note: Set the Center Freq phase value to the unwrapped value.
  note: Re-swap the data for display
  note: Unwrap requires frame based data
  IN : Inport  OutDataType=sfix(16)  OutScaling=2^0
  Add1 : Sum  Inputs=+-  OutDataType=sfix(16)  OutScaling=2^-10
  Array-Vector Add : dspmtrx3/Array-Vector Add  DialogController=dspDDGCreate  DialogControllerArgs=DataTag9  Dimension=2  V_Source=Input port  V_VectFromMask=[0.5 0.25]  firstCoeffDataTypeStr=Inherit: Same word length as input  firstCoeffLastDataTypeStr=Inherit: Same word length as input  firstCoeffMin=[]  firstCoeffMax=[]  outputDataTypeStr=Inherit: Same as accumulator  outputLastDataTypeStr=Inherit: Same as accumulator  outputMin=[]  outputMax=[]  roundingMode=Floor  overflowMode=off
  Constant : Constant  Value=[(ceil(NFFT*pcnt/200)):ceil(NFFT*pcnt/100) 1:ceil(NFFT*pcnt/200)-1];  OutDataType=sfix(16)  OutScaling=2^0
  Constant1 : Constant  Value=[(ceil(NFFT*pcnt/200)+1):ceil(NFFT*pcnt/100) 1:ceil(NFFT*pcnt/200)];  OutDataType=sfix(16)  OutScaling=2^0
  Frame Conversion : FrameConversion
  Frame Conversion3 : FrameConversion  OutFrame=Sample-based
  Unwrap : dspsigops/Unwrap  running=on  tol=pi
  Variable Selector : dspindex/Variable Selector  NumInputs=1  rowsOrCols=Rows  IdxMode=Variable  Elements=[1 3]  ZerOneIdxMode=One-based  errmode=Clip Index  FillMode=on  FillValues=0
  Variable Selector1 : dspindex/Variable Selector  NumInputs=1  rowsOrCols=Rows  IdxMode=Fixed  Elements=[1]  ZerOneIdxMode=One-based  errmode=Clip Index  FillMode=on  FillValues=0
  Variable Selector2 : dspindex/Variable Selector  NumInputs=1  rowsOrCols=Rows  IdxMode=Variable  Elements=[1 3]  ZerOneIdxMode=One-based  errmode=Clip Index  FillMode=on  FillValues=0
  Variable Selector4 : dspindex/Variable Selector  NumInputs=1  rowsOrCols=Rows  IdxMode=Fixed  Elements=length([(ceil(NFFT*pcnt/200)+1):ceil(NFFT*pcnt/100) 1:ceil(NFFT*pcnt/200)] )/2+1  ZerOneIdxMode=One-based  errmode=Clip Index  FillMode=on  FillValues=0
  Out1 : Outport  OutDataType=sfix(16)  OutScaling=2^0
  wires:
  Frame Conversion/1 -> Unwrap/1
  Variable Selector2/1 -> Out1/1
  IN/1 -> Variable Selector/1, Variable Selector1/1
  Constant/1 -> Variable Selector/2
  Variable Selector/1 -> Frame Conversion/1
  Variable Selector1/1 -> Add1/1
  Unwrap/1 -> Frame Conversion3/1
  Variable Selector4/1 -> Add1/2
  Constant1/1 -> Variable Selector2/2
  Frame Conversion3/1 -> Variable Selector4/1, Array-Vector Add/1
  Add1/1 -> Array-Vector Add/2
  Array-Vector Add/1 -> Variable Selector2/1
